simulink model "afe_abc_inv_psm"  (R2025a)
settings: Solver=ode1be  StartTime=0.0  StopTime=simlength  FixedStep=tc  MaxStep=tc
undefined symbols (not defined in the file): Adrso, Amplitude_U, Amplitude_V, Amplitude_W, Aresd, b, Bresd, Cresd, Crso, CTRPIFF_CLIP_RELEASE, dead_time_AFE, dead_time_INV, deepNEGeta, deepNEGxi, deepPOSxi, emf_fb_p, emf_fb_p_ccaller_1, emf_fb_p_ccaller_2, emf_p, emf_p_ccaller_1, emf_p_ccaller_2, end_time_LVRT, fPWM_AFE, fPWM_INV, g0_161Hz, g0_500Hz, g1_161Hz, g1_500Hz, i_grid_neg_eta_lim, i_grid_neg_eta_red_lim, i_grid_neg_xi_lim, i_grid_neg_xi_red_lim, i_grid_pos_eta_lim, i_grid_pos_eta_red_lim, ibez, id_lim, ieta_neg_ref_lim, ieta_pos_ref_lim, Igrid_phase_normalization_factor, iq_lim, ixi_pos_ref_lim, Jm, k_frt_ref, kg, ki_afe, ki_i, ki_rc_neg_grid, ki_rc_pos_grid, ki_vs, ki_w, kp_afe, kp_i, kp_rc_neg_grid, kp_rc_pos_grid, kp_vs, kp_w, kw, l1, l2, Ld_norm ... (+47)
libraries: fl_lib x121, nesl_utility x78, cstblocks x14, simulink x13, single_phase_transformer_lib x3, threephase_inductor_lib x2, flexshaft_lib x1, pmsm_uvw_with_harmonics_lib x1
(part 5 of 10)

== system afe_abc_inv_psm/afe_abc_inv_psm_mod1/afe_control/grid_current_sampling_and_alpha_beta_transformation/sample_hold_normalization ==
  ig_a : Inport
  ig_b : Inport  Port=2
  ig_c : Inport  Port=3
  Gain : Gain  Gain=1/Igrid_phase_normalization_factor
  Gain1 : Gain  Gain=1/Igrid_phase_normalization_factor
  Gain2 : Gain  Gain=1/Igrid_phase_normalization_factor
  Quantizer : Quantizer  QuantizationInterval=adc_quantization
  Quantizer1 : Quantizer  QuantizationInterval=adc_quantization
  Quantizer2 : Quantizer  QuantizationInterval=adc_quantization
  Unit Delay : UnitDelay  SampleTime=ts_afe  HasFrameUpgradeWarning=on
  Unit Delay1 : UnitDelay  SampleTime=ts_afe  HasFrameUpgradeWarning=on
  Unit Delay2 : UnitDelay  SampleTime=ts_afe  HasFrameUpgradeWarning=on
  Zero-Order Hold : ZeroOrderHold  SampleTime=ts_afe
  Zero-Order Hold1 : ZeroOrderHold  SampleTime=ts_afe
  Zero-Order Hold2 : ZeroOrderHold  SampleTime=ts_afe
  ig_a_pu : Outport
  ig_b_pu : Outport  Port=2
  ig_c_pu : Outport  Port=3
  wires:
  ig_a/1 -> Gain/1
  Zero-Order Hold/1 -> Unit Delay/1
  ig_c/1 -> Gain2/1
  ig_b/1 -> Gain1/1
  Unit Delay/1 -> ig_a_pu/1
  Unit Delay1/1 -> ig_b_pu/1
  Unit Delay2/1 -> ig_c_pu/1
  Zero-Order Hold1/1 -> Unit Delay1/1
  Zero-Order Hold2/1 -> Unit Delay2/1
  Quantizer/1 -> Zero-Order Hold/1
  Gain1/1 -> Quantizer1/1
  Gain2/1 -> Quantizer2/1
  Gain/1 -> Quantizer/1
  Quantizer1/1 -> Zero-Order Hold1/1
  Quantizer2/1 -> Zero-Order Hold2/1

== system afe_abc_inv_psm/afe_abc_inv_psm_mod1/afe_control/grid_voltage_phase_lock_loops/DDSRF-PLL ==
  pll_stageA : Subsystem
  pll_stageB : Subsystem
  gamma_grid_ddsrf_pll : Outport
  omega_grid_ddsrf_pll : Outport  Port=2
  wires:
  pll_stageB/1(gamma_grid_ddsrf_pll) -> pll_stageA/1(gamma_grid), gamma_grid_ddsrf_pll/1
  pll_stageA/2(u_grid_pos_eta) -> pll_stageB/2(u_grid_pos_eta)  "u_grid_pos_eta"
  pll_stageA/1(u_grid_pos_xi) -> pll_stageB/1(u_grid_pos_xi)  "u_grid_pos_xi"
  pll_stageB/2(omega_grid_ddsrf_pll) -> omega_grid_ddsrf_pll/1

== system afe_abc_inv_psm/afe_abc_inv_psm_mod1/afe_control/grid_voltage_phase_lock_loops/DQ-PLL ==
  pll_stageA : Subsystem
  pll_stageB : Subsystem
  gamma_grid_dqpll : Outport
  omega_grid_dqpll : Outport  Port=2
  wires:
  pll_stageA/2(u_grid_pos_eta) -> pll_stageB/2(u_grid_pos_eta)  "u_grid_pos_eta"
  pll_stageB/1(gamma_grid_dqpll) -> pll_stageA/1(gamma_grid), gamma_grid_dqpll/1
  pll_stageA/1(u_grid_pos_xi) -> pll_stageB/1(u_grid_pos_xi)  "u_grid_pos_xi"
  pll_stageB/2(omega_grid_dqpll) -> omega_grid_dqpll/1

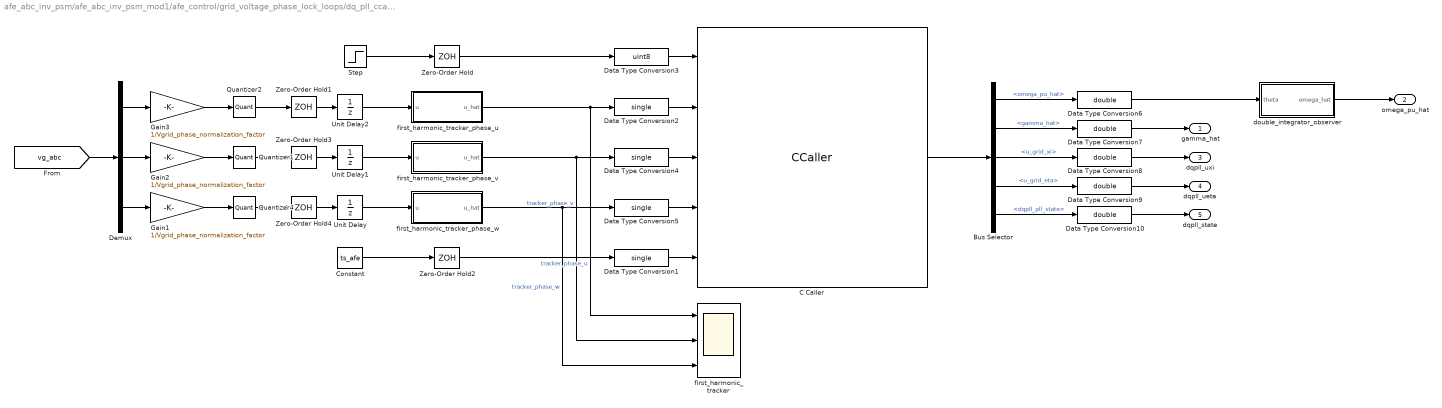
== system afe_abc_inv_psm/afe_abc_inv_psm_mod1/afe_control/grid_voltage_phase_lock_loops/dq_pll_ccaller ==
  Bus Selector : BusSelector  OutputSignals=omega_pu_hat,gamma_hat,u_grid_xi,u_grid_eta,dqpll_pll_state
  C Caller : CCaller  FunctionName=dqpll_grid_process_simulink  PortSpecificationStruct="%)30     .    N H   8    (     @         %    \"     8    !     0         %  0 \"0    $    _    07)G3F%M90  4&]R=$YA;64 4V-O<&4     26YD97@     5'EP90      4VEZ90      27-';&]B86P   X    P    !@    @    $          4    (     0    ,    !         !   P!O=70 #@   #     &    \"     0         !0    @    !     P    $         $  # &]U=  .    .     8    (    !          %    \"     $    &     0         0   ...(+3319 chars)"  SampleTime=ts_afe
  Constant : Constant  Value=ts_afe
  Data Type Conversion{1..2,4..5} (4 alike) : DataTypeConversion  OutDataTypeStr=single  SaturateOnIntegerOverflow=off  RndMeth=Floor
  Data Type Conversion{6..10} (5 alike) : DataTypeConversion  OutDataTypeStr=double  SaturateOnIntegerOverflow=off  RndMeth=Floor
  Data Type Conversion3 : DataTypeConversion  OutDataTypeStr=uint8  SaturateOnIntegerOverflow=off  RndMeth=Floor
  Demux : Demux  Outputs=3
  Gain1 : Gain  Gain=1/Vgrid_phase_normalization_factor
  Gain2 : Gain  Gain=1/Vgrid_phase_normalization_factor
  Gain3 : Gain  Gain=1/Vgrid_phase_normalization_factor
  Quantizer1 : Quantizer  QuantizationInterval=adc_quantization
  Quantizer2 : Quantizer  QuantizationInterval=adc_quantization
  Quantizer4 : Quantizer  QuantizationInterval=adc_quantization
  Step : Step  Time=0.01  Before=1  After=0  SampleTime=0
  Unit Delay : UnitDelay  SampleTime=ts_afe  HasFrameUpgradeWarning=on
  Unit Delay1 : UnitDelay  SampleTime=ts_afe  HasFrameUpgradeWarning=on
  Unit Delay2 : UnitDelay  SampleTime=ts_afe  HasFrameUpgradeWarning=on
  Zero-Order Hold : ZeroOrderHold  SampleTime=ts_afe
  Zero-Order Hold1 : ZeroOrderHold  SampleTime=-1
  Zero-Order Hold2 : ZeroOrderHold  SampleTime=ts_afe
  Zero-Order Hold3 : ZeroOrderHold  SampleTime=-1
  Zero-Order Hold4 : ZeroOrderHold  SampleTime=-1
  double_integrator_observer : Subsystem
  first_harmonic_tracker : Scope  NumInputPorts=3
      settings: SampleTime=ts_afe  ActiveDisplayYMinimum=-1.8038768619298935  ActiveDisplayYMaximum=1.5708545297384262
  first_harmonic_tracker_phase_u : Subsystem
  first_harmonic_tracker_phase_v : Subsystem
  first_harmonic_tracker_phase_w : Subsystem
  gamma_hat : Outport  VectorParamsAs1DForOutWhenUnconnected=off
  omega_pu_hat : Outport  Port=2  VectorParamsAs1DForOutWhenUnconnected=off
  dqpll_uxi : Outport  Port=3  VectorParamsAs1DForOutWhenUnconnected=off
  dqpll_ueta : Outport  Port=4  VectorParamsAs1DForOutWhenUnconnected=off
  dqpll_state : Outport  Port=5  VectorParamsAs1DForOutWhenUnconnected=off
  wires:
  Zero-Order Hold/1 -> Data Type Conversion3/1
  Step/1 -> Zero-Order Hold/1
  Zero-Order Hold2/1 -> Data Type Conversion1/1
  Constant/1 -> Zero-Order Hold2/1
  Data Type Conversion3/1 -> C Caller/1
  Data Type Conversion2/1 -> C Caller/2
  Data Type Conversion4/1 -> C Caller/3
  Data Type Conversion5/1 -> C Caller/4
  Data Type Conversion1/1 -> C Caller/5
  C Caller/1 -> Bus Selector/1
  Bus Selector/1 -> Data Type Conversion6/1  "<omega_pu_hat>"
  Bus Selector/2 -> Data Type Conversion7/1  "<gamma_hat>"
  Bus Selector/3 -> Data Type Conversion8/1  "<u_grid_xi>"
  Bus Selector/4 -> Data Type Conversion9/1  "<u_grid_eta>"
  Bus Selector/5 -> Data Type Conversion10/1  "<dqpll_pll_state>"
  Data Type Conversion6/1 -> double_integrator_observer/1(theta)
  Data Type Conversion7/1 -> gamma_hat/1
  Data Type Conversion10/1 -> dqpll_state/1
  Data Type Conversion8/1 -> dqpll_uxi/1
  Data Type Conversion9/1 -> dqpll_ueta/1
  [vg_abc] -> Demux/1
  Quantizer4/1 -> Zero-Order Hold4/1
  Quantizer2/1 -> Zero-Order Hold1/1
  Gain2/1 -> Quantizer1/1
  Gain3/1 -> Quantizer2/1
  Gain1/1 -> Quantizer4/1
  Zero-Order Hold1/1 -> Unit Delay2/1
  Unit Delay2/1 -> first_harmonic_tracker_phase_u/1(u)
  Demux/1 -> Gain3/1
  Unit Delay1/1 -> first_harmonic_tracker_phase_v/1(u)
  Demux/2 -> Gain2/1
  Demux/3 -> Gain1/1
  Unit Delay/1 -> first_harmonic_tracker_phase_w/1(u)
  Quantizer1/1 -> Zero-Order Hold3/1
  Zero-Order Hold3/1 -> Unit Delay1/1
  Zero-Order Hold4/1 -> Unit Delay/1
  double_integrator_observer/1(omega_hat) -> omega_pu_hat/1
  first_harmonic_tracker_phase_u/1(u_hat) -> first_harmonic_tracker/1, Data Type Conversion2/1  "tracker_phase_u"
  first_harmonic_tracker_phase_v/1(u_hat) -> first_harmonic_tracker/2, Data Type Conversion4/1  "tracker_phase_v"
  first_harmonic_tracker_phase_w/1(u_hat) -> first_harmonic_tracker/3, Data Type Conversion5/1  "tracker_phase_w"

== system afe_abc_inv_psm/afe_abc_inv_psm_mod1/afe_control/grid_voltage_sampling_and_alpha_beta_transformation/sample_hold_normalization ==
  vg_a : Inport
  vg_b : Inport  Port=2
  vg_c : Inport  Port=3
  Gain : Gain  Gain=1/Vgrid_phase_normalization_factor
  Gain1 : Gain  Gain=1/Vgrid_phase_normalization_factor
  Gain2 : Gain  Gain=1/Vgrid_phase_normalization_factor
  Quantizer1 : Quantizer  QuantizationInterval=adc_quantization
  Quantizer2 : Quantizer  QuantizationInterval=adc_quantization
  Quantizer3 : Quantizer  QuantizationInterval=adc_quantization
  Unit Delay : UnitDelay  SampleTime=ts_afe  HasFrameUpgradeWarning=on
  Unit Delay1 : UnitDelay  SampleTime=ts_afe  HasFrameUpgradeWarning=on
  Unit Delay2 : UnitDelay  SampleTime=ts_afe  HasFrameUpgradeWarning=on
  Zero-Order Hold : ZeroOrderHold  SampleTime=ts_afe
  Zero-Order Hold1 : ZeroOrderHold  SampleTime=ts_afe
  Zero-Order Hold2 : ZeroOrderHold  SampleTime=ts_afe
  vg_a_pu : Outport
  vg_b_pu : Outport  Port=2
  vg_c_pu : Outport  Port=3
  wires:
  vg_a/1 -> Gain/1
  Zero-Order Hold/1 -> Unit Delay/1
  vg_c/1 -> Gain2/1
  vg_b/1 -> Gain1/1
  Unit Delay/1 -> vg_a_pu/1
  Unit Delay1/1 -> vg_b_pu/1
  Unit Delay2/1 -> vg_c_pu/1
  Zero-Order Hold1/1 -> Unit Delay1/1
  Zero-Order Hold2/1 -> Unit Delay2/1
  Quantizer1/1 -> Zero-Order Hold/1
  Gain1/1 -> Quantizer2/1
  Gain2/1 -> Quantizer3/1
  Gain/1 -> Quantizer1/1
  Quantizer2/1 -> Zero-Order Hold1/1
  Quantizer3/1 -> Zero-Order Hold2/1

== system afe_abc_inv_psm/afe_abc_inv_psm_mod1/afe_control/islanding_mode_detector/Moving Average Filter ==
  u_7th : Inport
  In3 : Inport  Port=2
  Bus Selector : BusSelector  OutputSignals=ts,sshort,slong,pinput,cbpointer,cbsample,mavg_output
  C Caller : CCaller  FunctionName=mavgflt_process_simulink  PortSpecificationStruct="%)30     .    B H   8    (     @         %    \"     8    !     0         %  0 \"0    $    _    07)G3F%M90  4&]R=$YA;64 4V-O<&4     26YD97@     5'EP90      4VEZ90      27-';&]B86P   X    P    !@    @    $          4    (     0    ,    !         !   P!O=70 #@   #     &    \"     0         !0    @    !     P    $         $  # &]U=  .    .     8    (    !          %    \"     $    &     0         0   ...(+3251 chars)"  SampleTime=ts_afe
  Compare To Zero : simulink/Logic and Bit Operations/Compare To Zero  relop=>  OutDataTypeStr=boolean
  Constant : Constant  Value=9
  Constant5 : Constant  Value=ts_afe
  Data Type Conversion : DataTypeConversion  OutDataTypeStr=single  SaturateOnIntegerOverflow=off  RndMeth=Floor
  Data Type Conversion1 : DataTypeConversion  OutDataTypeStr=single  SaturateOnIntegerOverflow=off  RndMeth=Floor
  Data Type Conversion2 : DataTypeConversion  OutDataTypeStr=single  SaturateOnIntegerOverflow=off  RndMeth=Floor
  Data Type Conversion3 : DataTypeConversion  OutDataTypeStr=double  SaturateOnIntegerOverflow=off  RndMeth=Floor
  Data Type Conversion4 : DataTypeConversion  OutDataTypeStr=uint8  SaturateOnIntegerOverflow=off  RndMeth=Floor
  Data Type Conversion5 : DataTypeConversion  OutDataTypeStr=uint8  SaturateOnIntegerOverflow=off  RndMeth=Floor
  Enabled Subsystem : Subsystem  TreatAsAtomicUnit=on
  Reset Trigger : Subsystem
  Terminator{,1..5} (6 alike) : Terminator
  Zero-Order Hold1 : ZeroOrderHold  SampleTime=ts_afe
  Zero-Order Hold2 : ZeroOrderHold  SampleTime=ts_afe
  xi : Outport
  wires:
  Bus Selector/5 -> Terminator2/1  "<cbpointer>"
  Bus Selector/4 -> Terminator1/1  "<pinput>"
  Data Type Conversion3/1 -> xi/1  "output"
  Zero-Order Hold2/1 -> Data Type Conversion/1  "d1"
  Enabled Subsystem/1(Out1) -> Data Type Conversion1/1
  Compare To Zero/1 -> Enabled Subsystem/Enable
  In3/1 -> Enabled Subsystem/1(In1), Compare To Zero/1  "omega_grid"
  Constant5/1 -> Zero-Order Hold1/1
  Zero-Order Hold1/1 -> Data Type Conversion2/1  "d1"
  Bus Selector/3 -> Terminator4/1  "<slong>"
  Bus Selector/2 -> Terminator3/1  "<sshort>"
  Bus Selector/1 -> Terminator/1  "<ts>"
  C Caller/1 -> Bus Selector/1  "out"
  u_7th/1 -> Zero-Order Hold2/1  "input"
  Data Type Conversion4/1 -> C Caller/5
  Data Type Conversion/1 -> C Caller/1  "input"
  Data Type Conversion5/1 -> C Caller/4
  Data Type Conversion2/1 -> C Caller/3
  Data Type Conversion1/1 -> C Caller/2
  Reset Trigger/1(Out1) -> Data Type Conversion5/1
  Constant/1 -> Data Type Conversion4/1
  Bus Selector/6 -> Terminator5/1  "<cbsample>"
  Bus Selector/7 -> Data Type Conversion3/1  "<mavg_output>"

== system afe_abc_inv_psm/afe_abc_inv_psm_mod1/afe_control/islanding_mode_detector/Moving Average Filter1 ==
  u_7th : Inport
  In3 : Inport  Port=2
  Bus Selector : BusSelector  OutputSignals=ts,sshort,slong,pinput,cbpointer,cbsample,mavg_output
  C Caller : CCaller  FunctionName=mavgflt_process_simulink  PortSpecificationStruct="%)30     .    B H   8    (     @         %    \"     8    !     0         %  0 \"0    $    _    07)G3F%M90  4&]R=$YA;64 4V-O<&4     26YD97@     5'EP90      4VEZ90      27-';&]B86P   X    P    !@    @    $          4    (     0    ,    !         !   P!O=70 #@   #     &    \"     0         !0    @    !     P    $         $  # &]U=  .    .     8    (    !          %    \"     $    &     0         0   ...(+3251 chars)"  SampleTime=ts_afe
  Compare To Zero : simulink/Logic and Bit Operations/Compare To Zero  relop=>  OutDataTypeStr=boolean
  Constant : Constant  Value=10
  Constant5 : Constant  Value=ts_afe
  Data Type Conversion : DataTypeConversion  OutDataTypeStr=single  SaturateOnIntegerOverflow=off  RndMeth=Floor
  Data Type Conversion1 : DataTypeConversion  OutDataTypeStr=single  SaturateOnIntegerOverflow=off  RndMeth=Floor
  Data Type Conversion2 : DataTypeConversion  OutDataTypeStr=single  SaturateOnIntegerOverflow=off  RndMeth=Floor
  Data Type Conversion3 : DataTypeConversion  OutDataTypeStr=double  SaturateOnIntegerOverflow=off  RndMeth=Floor
  Data Type Conversion4 : DataTypeConversion  OutDataTypeStr=uint8  SaturateOnIntegerOverflow=off  RndMeth=Floor
  Data Type Conversion5 : DataTypeConversion  OutDataTypeStr=uint8  SaturateOnIntegerOverflow=off  RndMeth=Floor
  Enabled Subsystem : Subsystem  TreatAsAtomicUnit=on
  Reset Trigger : Subsystem
  Terminator{,1..5} (6 alike) : Terminator
  Zero-Order Hold1 : ZeroOrderHold  SampleTime=ts_afe
  Zero-Order Hold2 : ZeroOrderHold  SampleTime=ts_afe
  xi : Outport
  wires:
  Bus Selector/7 -> Data Type Conversion3/1  "<mavg_output>"
  Bus Selector/6 -> Terminator5/1  "<cbsample>"
  Constant/1 -> Data Type Conversion4/1
  Reset Trigger/1(Out1) -> Data Type Conversion5/1
  Data Type Conversion1/1 -> C Caller/2
  Data Type Conversion2/1 -> C Caller/3
  Data Type Conversion5/1 -> C Caller/4
  Data Type Conversion/1 -> C Caller/1  "input"
  Data Type Conversion4/1 -> C Caller/5
  u_7th/1 -> Zero-Order Hold2/1  "input"
  C Caller/1 -> Bus Selector/1  "out"
  Bus Selector/1 -> Terminator/1  "<ts>"
  Bus Selector/2 -> Terminator3/1  "<sshort>"
  Bus Selector/3 -> Terminator4/1  "<slong>"
  Zero-Order Hold1/1 -> Data Type Conversion2/1  "d1"
  Constant5/1 -> Zero-Order Hold1/1
  In3/1 -> Compare To Zero/1, Enabled Subsystem/1(In1)  "omega_grid"
  Compare To Zero/1 -> Enabled Subsystem/Enable
  Enabled Subsystem/1(Out1) -> Data Type Conversion1/1
  Zero-Order Hold2/1 -> Data Type Conversion/1  "d1"
  Data Type Conversion3/1 -> xi/1  "output"
  Bus Selector/4 -> Terminator1/1  "<pinput>"
  Bus Selector/5 -> Terminator2/1  "<cbpointer>"

== system afe_abc_inv_psm/afe_abc_inv_psm_mod1/afe_control/sequences_current_control/Negative-Seq. eta-Control ==
  ff : Inport
  e : Inport  Port=2
  1/Ti : Gain  Gain=kp_rc_neg_grid  SaturateOnIntegerOverflow=on  OutDataTypeStr=Inherit: Same as input  ParamDataTypeStr=Inherit: Same as input
  1/Ti1 : Gain  SaturateOnIntegerOverflow=on  OutDataTypeStr=Inherit: Same as input  ParamDataTypeStr=Inherit: Same as input
  Saturation : Saturate  UpperLimit=ieta_neg_ref_lim  LowerLimit=-ieta_neg_ref_lim
  Sum : Sum  Inputs=|++
  Sum2 : Sum  Inputs=+++  SaturateOnIntegerOverflow=on
  Sum3 : Sum  Inputs=-+  SaturateOnIntegerOverflow=on
  Unit Delay4 : UnitDelay  SampleTime=ts_afe  HasFrameUpgradeWarning=on
  kp : Gain  Gain=ki_rc_neg_grid*ts_afe  SaturateOnIntegerOverflow=on  OutDataTypeStr=Inherit: Same as input  ParamDataTypeStr=Inherit: Same as input
  u : Outport  VectorParamsAs1DForOutWhenUnconnected=off
  wires:
  Unit Delay4/1 -> Sum2/3
  Sum3/1 -> Unit Delay4/1
  kp/1 -> Sum2/2
  Sum2/1 -> Saturation/1
  1/Ti/1 -> Sum2/1, Sum3/1
  Saturation/1 -> Sum/1, Sum3/2
  Sum/1 -> u/1
  ff/1 -> 1/Ti1/1
  1/Ti1/1 -> Sum/2
  e/1 -> 1/Ti/1, kp/1  "e"

== system afe_abc_inv_psm/afe_abc_inv_psm_mod1/afe_control/sequences_current_control/Negative-Seq. xi-Control ==
  ff : Inport
  e : Inport  Port=2
  1/Ti : Gain  Gain=kp_rc_neg_grid  SaturateOnIntegerOverflow=on  OutDataTypeStr=Inherit: Same as input  ParamDataTypeStr=Inherit: Same as input
  1/Ti1 : Gain  SaturateOnIntegerOverflow=on  OutDataTypeStr=Inherit: Same as input  ParamDataTypeStr=Inherit: Same as input
  Saturation : Saturate  UpperLimit=ieta_pos_ref_lim  LowerLimit=-ieta_pos_ref_lim
  Sum : Sum  Inputs=|++
  Sum2 : Sum  Inputs=+++  SaturateOnIntegerOverflow=on
  Sum3 : Sum  Inputs=-+  SaturateOnIntegerOverflow=on
  Unit Delay4 : UnitDelay  SampleTime=ts_afe  HasFrameUpgradeWarning=on
  kp : Gain  Gain=ki_rc_neg_grid*ts_afe  SaturateOnIntegerOverflow=on  OutDataTypeStr=Inherit: Same as input  ParamDataTypeStr=Inherit: Same as input
  u : Outport  VectorParamsAs1DForOutWhenUnconnected=off
  wires:
  Unit Delay4/1 -> Sum2/3
  Sum3/1 -> Unit Delay4/1
  kp/1 -> Sum2/2
  Sum2/1 -> Saturation/1
  1/Ti/1 -> Sum2/1, Sum3/1
  Saturation/1 -> Sum/1, Sum3/2
  Sum/1 -> u/1
  ff/1 -> 1/Ti1/1
  1/Ti1/1 -> Sum/2
  e/1 -> 1/Ti/1, kp/1  "e"

== system afe_abc_inv_psm/afe_abc_inv_psm_mod1/afe_control/sequences_current_control/Positive-Seq. eta-Control ==
  ff : Inport
  e : Inport  Port=2
  1/Ti : Gain  Gain=kp_rc_pos_grid  SaturateOnIntegerOverflow=on  OutDataTypeStr=Inherit: Same as input  ParamDataTypeStr=Inherit: Same as input
  1/Ti1 : Gain  SaturateOnIntegerOverflow=on  OutDataTypeStr=Inherit: Same as input  ParamDataTypeStr=Inherit: Same as input
  Saturation : Saturate  UpperLimit=ieta_pos_ref_lim  LowerLimit=-ieta_pos_ref_lim
  Sum : Sum  Inputs=|++
  Sum2 : Sum  Inputs=+++  SaturateOnIntegerOverflow=on
  Sum3 : Sum  Inputs=-+  SaturateOnIntegerOverflow=on
  Unit Delay4 : UnitDelay  SampleTime=ts_afe  HasFrameUpgradeWarning=on
  kp : Gain  Gain=ki_rc_pos_grid*ts_afe  SaturateOnIntegerOverflow=on  OutDataTypeStr=Inherit: Same as input  ParamDataTypeStr=Inherit: Same as input
  u : Outport  VectorParamsAs1DForOutWhenUnconnected=off
  wires:
  Unit Delay4/1 -> Sum2/3
  Sum3/1 -> Unit Delay4/1
  kp/1 -> Sum2/2
  Sum2/1 -> Saturation/1
  1/Ti/1 -> Sum2/1, Sum3/1
  Saturation/1 -> Sum/1, Sum3/2
  Sum/1 -> u/1
  ff/1 -> 1/Ti1/1
  1/Ti1/1 -> Sum/2
  e/1 -> 1/Ti/1, kp/1  "e"

== system afe_abc_inv_psm/afe_abc_inv_psm_mod1/afe_control/voltage_sequence_avg/average_filter_ccaller ==
  v_grid_pos_xi : Inport
  v_grid_pos_eta : Inport  Port=2
  v_grid_neg_xi : Inport  Port=3
  v_grid_neg_eta : Inport  Port=4
  Moving Average Filter1 : Subsystem
  Moving Average Filter2 : Subsystem
  Moving Average Filter3 : Subsystem
  Moving Average Filter4 : Subsystem
  v_grid_pos_xi_avg : Outport
  v_grid_pos_eta_avg : Outport  Port=2
  v_grid_neg_xi_avg : Outport  Port=3
  v_grid_neg_eta_avg : Outport  Port=4
  wires:
  Moving Average Filter2/1(xi) -> v_grid_pos_eta_avg/1
  [omega_grid_pll] -> Moving Average Filter1/2(In3), Moving Average Filter2/2(In3), Moving Average Filter4/2(In3), Moving Average Filter3/2(In3)
  v_grid_pos_xi/1 -> Moving Average Filter1/1(In2)
  v_grid_neg_xi/1 -> Moving Average Filter3/1(In2)
  v_grid_neg_eta/1 -> Moving Average Filter4/1(In2)
  Moving Average Filter3/1(xi) -> v_grid_neg_xi_avg/1
  Moving Average Filter4/1(xi) -> v_grid_neg_eta_avg/1
  Moving Average Filter1/1(xi) -> v_grid_pos_xi_avg/1
  v_grid_pos_eta/1 -> Moving Average Filter2/1(In2)

== system afe_abc_inv_psm/afe_abc_inv_psm_mod1/afe_control/voltage_sequence_avg/average_filter_simulink ==
  v_grid_pos_xi : Inport
  v_grid_pos_eta : Inport  Port=2
  v_grid_neg_xi : Inport  Port=3
  v_grid_neg_eta : Inport  Port=4
  mavg_1 : Subsystem
  mavg_2 : Subsystem
  mavg_3 : Subsystem
  mavg_4 : Subsystem
  v_grid_pos_xi_avg : Outport
  v_grid_pos_eta_avg : Outport  Port=2
  v_grid_neg_xi_avg : Outport  Port=3
  v_grid_neg_eta_avg : Outport  Port=4
  wires:
  mavg_3/1(out) -> v_grid_neg_xi_avg/1
  mavg_1/1(out) -> v_grid_pos_xi_avg/1
  v_grid_pos_eta/1 -> mavg_2/1(in)
  v_grid_neg_eta/1 -> mavg_4/1(in)
  v_grid_pos_xi/1 -> mavg_1/1(in)
  mavg_4/1(out) -> v_grid_neg_eta_avg/1
  v_grid_neg_xi/1 -> mavg_3/1(in)
  mavg_2/1(out) -> v_grid_pos_eta_avg/1

== system afe_abc_inv_psm/afe_abc_inv_psm_mod1/inverter/inverter/sv_pwm ==
  ab : Inport
  enable : Inport  Port=2
  Bus Selector : BusSelector  OutputSignals=da,db,dc
  Bus Selector1 : BusSelector  OutputSignals=ua,ub
  C Caller : CCaller  FunctionName=sv_pwm_process_simulink  PortSpecificationStruct="%)30     .    V @   8    (     @         %    \"     4    !     0         %  0 \"0    $    _    07)G3F%M90  4&]R=$YA;64 4V-O<&4     26YD97@     5'EP90      4VEZ90      27-';&]B86P   X    P    !@    @    $          4    (     0    ,    !         !   P!O=70 #@   #     &    \"     0         !0    @    !     P    $         $  # &]U=  .    .     8    (    !          %    \"     $    &     0         0   ...(+2669 chars)"  SampleTime=ts_inv
  Constant : Constant  Value=ts_inv
  Data Type Conversion1 : DataTypeConversion  OutDataTypeStr=double  SaturateOnIntegerOverflow=off  RndMeth=Floor
  Data Type Conversion15 : DataTypeConversion  OutDataTypeStr=single  SaturateOnIntegerOverflow=off  RndMeth=Floor
  Data Type Conversion16 : DataTypeConversion  OutDataTypeStr=single  SaturateOnIntegerOverflow=off  RndMeth=Floor
  Data Type Conversion17 : DataTypeConversion  OutDataTypeStr=uint32  SaturateOnIntegerOverflow=off  RndMeth=Floor
  Data Type Conversion18 : DataTypeConversion  OutDataTypeStr=single  SaturateOnIntegerOverflow=off  RndMeth=Floor
  Data Type Conversion2 : DataTypeConversion  OutDataTypeStr=double  SaturateOnIntegerOverflow=off  RndMeth=Floor
  Data Type Conversion3 : DataTypeConversion  OutDataTypeStr=double  SaturateOnIntegerOverflow=off  RndMeth=Floor
  Zero-Order Hold{,1..3} (4 alike) : ZeroOrderHold  SampleTime=ts_afe
  modulator1 : Subsystem
  firing_gates : Outport
  wires:
  Data Type Conversion1/1 -> modulator1/1(u)  "du"
  Zero-Order Hold/1 -> C Caller/1
  Zero-Order Hold2/1 -> C Caller/3
  Constant/1 -> Data Type Conversion16/1
  Data Type Conversion18/1 -> Zero-Order Hold/1
  enable/1 -> Data Type Conversion17/1
  Data Type Conversion2/1 -> modulator1/2(v)  "dv"
  Data Type Conversion16/1 -> Zero-Order Hold2/1
  Zero-Order Hold1/1 -> C Caller/2
  Data Type Conversion17/1 -> Zero-Order Hold3/1
  Zero-Order Hold3/1 -> C Caller/4
  Data Type Conversion15/1 -> Zero-Order Hold1/1
  C Caller/1 -> Bus Selector/1  "out"
  Data Type Conversion3/1 -> modulator1/3(w)  "dw"
  modulator1/1(cmd_gates) -> firing_gates/1
  ab/1 -> Bus Selector1/1
  Bus Selector1/1 -> Data Type Conversion18/1  "<ua>"
  Bus Selector1/2 -> Data Type Conversion15/1  "<ub>"
  Bus Selector/1 -> Data Type Conversion1/1  "<da>"
  Bus Selector/3 -> Data Type Conversion3/1  "<dc>"
  Bus Selector/2 -> Data Type Conversion2/1  "<db>"

== system afe_abc_inv_psm/afe_abc_inv_psm_mod1/inverter/inverter/switch_1 ==
  Diode : fl_lib/Electrical/Electrical Elements/Diode  Vf=Vgamma V  Ron=Ron Ohm  Goff=1e-8 1/Ohm  i_specify=off  i_priority=None  i=0 A  i_nominal_specify=off  i_nominal_value=1  i_nominal_unit=A  v_specify=off  v_priority=None  v=0 V  v_nominal_specify=off  v_nominal_value=1  v_nominal_unit=V
  Switch : fl_lib/Electrical/Electrical Elements/Switch  R_closed=Ron Ohm  G_open=1e-8 1/Ohm  Threshold=7.5  i_specify=off  i_priority=None  i=0 A  i_nominal_specify=off  i_nominal_value=1  i_nominal_unit=A  v_specify=off  v_priority=None  v=0 V  v_nominal_specify=off  v_nominal_value=1  v_nominal_unit=V
  G : PMIOPort  Side=Left
  C : PMIOPort  Port=2  Side=Left
  E : PMIOPort  Port=3  Side=Right
  connections:
  Switch/RConn2 -- C/RConn1 -- Diode/RConn1
  Switch/RConn1 -- G/RConn1
  Switch/LConn1 -- E/RConn1 -- Diode/LConn1

== system afe_abc_inv_psm/afe_abc_inv_psm_mod1/inverter/inverter/switch_2 ==
  Diode : fl_lib/Electrical/Electrical Elements/Diode  Vf=Vgamma V  Ron=Ron Ohm  Goff=1e-8 1/Ohm  i_specify=off  i_priority=None  i=0 A  i_nominal_specify=off  i_nominal_value=1  i_nominal_unit=A  v_specify=off  v_priority=None  v=0 V  v_nominal_specify=off  v_nominal_value=1  v_nominal_unit=V
  Switch : fl_lib/Electrical/Electrical Elements/Switch  R_closed=Ron Ohm  G_open=1e-8 1/Ohm  Threshold=7.5  i_specify=off  i_priority=None  i=0 A  i_nominal_specify=off  i_nominal_value=1  i_nominal_unit=A  v_specify=off  v_priority=None  v=0 V  v_nominal_specify=off  v_nominal_value=1  v_nominal_unit=V
  G : PMIOPort  Side=Left
  C : PMIOPort  Port=2  Side=Left
  E : PMIOPort  Port=3  Side=Right
  connections:
  Diode/LConn1 -- E/RConn1 -- Switch/LConn1
  Switch/RConn1 -- G/RConn1
  Diode/RConn1 -- C/RConn1 -- Switch/RConn2

== system afe_abc_inv_psm/afe_abc_inv_psm_mod1/inverter/inverter/switch_3 ==
  Diode : fl_lib/Electrical/Electrical Elements/Diode  Vf=Vgamma V  Ron=Ron Ohm  Goff=1e-8 1/Ohm  i_specify=off  i_priority=None  i=0 A  i_nominal_specify=off  i_nominal_value=1  i_nominal_unit=A  v_specify=off  v_priority=None  v=0 V  v_nominal_specify=off  v_nominal_value=1  v_nominal_unit=V
  Switch : fl_lib/Electrical/Electrical Elements/Switch  R_closed=Ron Ohm  G_open=1e-8 1/Ohm  Threshold=7.5  i_specify=off  i_priority=None  i=0 A  i_nominal_specify=off  i_nominal_value=1  i_nominal_unit=A  v_specify=off  v_priority=None  v=0 V  v_nominal_specify=off  v_nominal_value=1  v_nominal_unit=V
  G : PMIOPort  Side=Left
  C : PMIOPort  Port=2  Side=Left
  E : PMIOPort  Port=3  Side=Right
  connections:
  Diode/LConn1 -- E/RConn1 -- Switch/LConn1
  Switch/RConn1 -- G/RConn1
  Diode/RConn1 -- C/RConn1 -- Switch/RConn2

== system afe_abc_inv_psm/afe_abc_inv_psm_mod1/inverter/inverter/switch_4 ==
  Diode : fl_lib/Electrical/Electrical Elements/Diode  Vf=Vgamma V  Ron=Ron Ohm  Goff=1e-8 1/Ohm  i_specify=off  i_priority=None  i=0 A  i_nominal_specify=off  i_nominal_value=1  i_nominal_unit=A  v_specify=off  v_priority=None  v=0 V  v_nominal_specify=off  v_nominal_value=1  v_nominal_unit=V
  Switch : fl_lib/Electrical/Electrical Elements/Switch  R_closed=Ron Ohm  G_open=1e-8 1/Ohm  Threshold=7.5  i_specify=off  i_priority=None  i=0 A  i_nominal_specify=off  i_nominal_value=1  i_nominal_unit=A  v_specify=off  v_priority=None  v=0 V  v_nominal_specify=off  v_nominal_value=1  v_nominal_unit=V
  G : PMIOPort  Side=Left
  C : PMIOPort  Port=2  Side=Left
  E : PMIOPort  Port=3  Side=Right
  connections:
  Switch/RConn2 -- C/RConn1 -- Diode/RConn1
  Switch/RConn1 -- G/RConn1
  Switch/LConn1 -- E/RConn1 -- Diode/LConn1

== system afe_abc_inv_psm/afe_abc_inv_psm_mod1/inverter/inverter/switch_5 ==
  Diode : fl_lib/Electrical/Electrical Elements/Diode  Vf=Vgamma V  Ron=Ron Ohm  Goff=1e-8 1/Ohm  i_specify=off  i_priority=None  i=0 A  i_nominal_specify=off  i_nominal_value=1  i_nominal_unit=A  v_specify=off  v_priority=None  v=0 V  v_nominal_specify=off  v_nominal_value=1  v_nominal_unit=V
  Switch : fl_lib/Electrical/Electrical Elements/Switch  R_closed=Ron Ohm  G_open=1e-8 1/Ohm  Threshold=7.5  i_specify=off  i_priority=None  i=0 A  i_nominal_specify=off  i_nominal_value=1  i_nominal_unit=A  v_specify=off  v_priority=None  v=0 V  v_nominal_specify=off  v_nominal_value=1  v_nominal_unit=V
  G : PMIOPort  Side=Left
  C : PMIOPort  Port=2  Side=Left
  E : PMIOPort  Port=3  Side=Right
  connections:
  Diode/LConn1 -- E/RConn1 -- Switch/LConn1
  Switch/RConn1 -- G/RConn1
  Diode/RConn1 -- C/RConn1 -- Switch/RConn2

== system afe_abc_inv_psm/afe_abc_inv_psm_mod1/inverter/inverter/switch_6 ==
  Diode : fl_lib/Electrical/Electrical Elements/Diode  Vf=Vgamma V  Ron=Ron Ohm  Goff=1e-8 1/Ohm  i_specify=off  i_priority=None  i=0 A  i_nominal_specify=off  i_nominal_value=1  i_nominal_unit=A  v_specify=off  v_priority=None  v=0 V  v_nominal_specify=off  v_nominal_value=1  v_nominal_unit=V
  Switch : fl_lib/Electrical/Electrical Elements/Switch  R_closed=Ron Ohm  G_open=1e-8 1/Ohm  Threshold=7.5  i_specify=off  i_priority=None  i=0 A  i_nominal_specify=off  i_nominal_value=1  i_nominal_unit=A  v_specify=off  v_priority=None  v=0 V  v_nominal_specify=off  v_nominal_value=1  v_nominal_unit=V
  G : PMIOPort  Side=Left
  C : PMIOPort  Port=2  Side=Left
  E : PMIOPort  Port=3  Side=Right
  connections:
  Switch/RConn2 -- C/RConn1 -- Diode/RConn1
  Switch/RConn1 -- G/RConn1
  Switch/LConn1 -- E/RConn1 -- Diode/LConn1

== system afe_abc_inv_psm/afe_abc_inv_psm_mod1/inverter_control/current_ctrl/bemf_observer ==
  ialpha_pu : Inport
  ibeta_pu : Inport  Port=2
  ualpha_pu : Inport  Port=3
  ubeta_pu : Inport  Port=4
  BEMF Observer simulink/Ccaller : Scope  NumInputPorts=2
      settings: SampleTime=tc  ActiveDisplayYMinimum=-1.1712299957043022  ActiveDisplayYMaximum=1.2529884353188021
  Mux : Mux  Inputs=3
  Mux1 : Mux  Inputs=3
  Variant Source : VariantSource  VariantControls={use_observer_from_simulink_module_1 == 1, use_observer_from_ccaller_module_1 == 1}
  Variant Source1 : VariantSource  VariantControls={use_observer_from_simulink_module_1 == 1, use_observer_from_ccaller_module_1 == 1}
  bemf_observer : Subsystem
  bemf_observer_ccaller : Subsystem
  double_integrator_observer : Subsystem
  phase_fault : Subsystem
  tag scope: omega_hat_pu=global, theta_hat=global
  wires:
  ialpha_pu/1 -> bemf_observer/1(ialpha_pu), bemf_observer_ccaller/1(ialpha_pu)
  ibeta_pu/1 -> bemf_observer/2(ibeta_pu), bemf_observer_ccaller/2(ibeta_pu)
  Mux/1 -> BEMF Observer simulink/Ccaller/1
  Mux1/1 -> BEMF Observer simulink/Ccaller/2
  double_integrator_observer/1(omega_pu_hat) -> Mux/3  "omega_pu_encoder"
  ualpha_pu/1 -> bemf_observer/3(ualpha_pu), bemf_observer_ccaller/3(ualpha_pu)
  ubeta_pu/1 -> bemf_observer/4(ubeta_pu), bemf_observer_ccaller/4(ubeta_pu)
  double_integrator_observer/2(theta_hat) -> Mux1/3  "theta_hat_encoder"
  [theta_elec_pmsm] -> phase_fault/1(theta_pmsm)  "theta_pmsm"
  phase_fault/1(theta) -> double_integrator_observer/1(theta)
  bemf_observer/1(omega_pu) -> Mux/1, Variant Source/1  "omega_pu"
  bemf_observer_ccaller/2(theta_hat) -> Mux1/2, Variant Source1/2  "theta_hat_code"
  bemf_observer_ccaller/1(omega_pu) -> Mux/2, Variant Source/2  "omega_pu_code"
  bemf_observer/2(theta_hat) -> Variant Source1/1, Mux1/1  "theta_hat"
  Variant Source1/1 -> [theta_hat]
  Variant Source/1 -> [omega_hat_pu]

== system afe_abc_inv_psm/afe_abc_inv_psm_mod1/inverter_control/current_ctrl/current_ctrl ==
  iq_ref : Inport
  MTPA : Subsystem
  Sqrt : Sqrt
  Square : Math  Operator=square
  Square1 : Math  Operator=square
  Sum : Sum  Inputs=|++
  To Workspace1 : ToWorkspace  VariableName=id_pu_sim  SampleTime=ts_inv
      settings: MaxDataPoints=Ns_inv
  To Workspace2 : ToWorkspace  VariableName=iq_pu_sim  SampleTime=ts_inv
      settings: MaxDataPoints=Ns_inv
  To Workspace3 : ToWorkspace  VariableName=id_ref_pu_sim  SampleTime=ts_inv
      settings: MaxDataPoints=Ns_inv
  To Workspace4 : ToWorkspace  VariableName=iq_ref_pu_sim  SampleTime=ts_inv
      settings: MaxDataPoints=Ns_inv
  To Workspace5 : ToWorkspace  VariableName=ud_pu_sim  SampleTime=ts_inv
      settings: MaxDataPoints=Ns_inv
  To Workspace6 : ToWorkspace  VariableName=uq_pu_sim  SampleTime=ts_inv
      settings: MaxDataPoints=Ns_inv
  To Workspace7 : ToWorkspace  VariableName=u_mot_pu_sim  SampleTime=ts_inv
      settings: MaxDataPoints=Ns_inv
  dq_pi_with_vector_antiwindup : Subsystem
  id_ref : Subsystem
      settings: PortSchema="{\"entries\":[{\"content\":{\"sides\":[{\"content\":{},\"type\":\"ConnectorPlacement.EquallySpacedRectSide\",\"uuid\":\"42af5d69-f0eb-42c6-9e03-28c1d0757323\"},{\"content\":{\"connectorIds\":[\"Out1\"],\"side\":\"RIGHT\"},\"type\":\"ConnectorPlacement.EquallySpacedRectSide\",\"uuid\":\"dd68a9f9-d15f-4e57-9d9e-130889a7b90c\"},{\"content\":{\"connectorIds\":[\"In1\"],\"side\":\"TOP\"},\"type\":\"ConnectorPlacement.EquallySpacedRectSide\",\"uuid\":\"68c797a2-8439-4b8d-8368-b7485adf0676\"}]},\"type\":\"ConnectorPlacement.EquallySpacedConnector\",\"uuid\":\"693c5f1c-0580-4626-8f13-b27865dfb3ac\"}],\"packageUris\":[\"http://schema.mathworks.com/mf0/Connector/R2020b\"],\"version\":\"1.0\"}"
  idref/id : Scope  NumInputPorts=2
      settings: SampleTime=tc  ActiveDisplayYMinimum=-0.5383825399353187  ActiveDisplayYMaximum=0.059820282309629005
  iqref/iq : Scope  NumInputPorts=2
      settings: SampleTime=tc  ActiveDisplayYMinimum=-1.1641617765003931  ActiveDisplayYMaximum=0.12935130850004364  DataLoggingVariableName=ScopeData2
  ud : Outport
  uq : Outport  Port=2
  tag scope: id_pu_ref=global, iq_pu_ref=global, u_mot_pu_sim=global, ud_pu_sim=global, uq_pu_sim=global
  wires:
  [iq_pu] -> To Workspace2/1, iqref/iq/2, dq_pi_with_vector_antiwindup/4(iq)  "iq"
  [id_pu] -> To Workspace1/1, idref/id/2, dq_pi_with_vector_antiwindup/2(id)  "id"
  MTPA/1(Id_ref_mtpa) -> id_ref/1(id_mtpa), [id_pu_ref]  "id_ref"
  iq_ref/1 -> MTPA/1(iq_ref), To Workspace4/1, iqref/iq/1, dq_pi_with_vector_antiwindup/3(iq_ref), [iq_pu_ref]  "iq_ref"
  dq_pi_with_vector_antiwindup/1(ctrl_d_u) -> To Workspace5/1, [ud_pu_sim], Square1/1, ud/1
  dq_pi_with_vector_antiwindup/2(ctrl_q_u) -> [uq_pu_sim], To Workspace6/1, Square/1, uq/1
  Square/1 -> Sum/1
  Sum/1 -> Sqrt/1
  Square1/1 -> Sum/2
  Sqrt/1 -> [u_mot_pu_sim], To Workspace7/1
  id_ref/1(id_ref) -> To Workspace3/1, dq_pi_with_vector_antiwindup/1(id_ref), idref/id/1

== system afe_abc_inv_psm/afe_abc_inv_psm_mod1/inverter_control/current_ctrl/current_transformation ==
  u : Inport
  v : Inport  Port=2
  w : Inport  Port=3
  To Workspace2 : ToWorkspace  VariableName=ialpha_pu_sim  SampleTime=ts_inv
      settings: MaxDataPoints=Ns_inv
  To Workspace3 : ToWorkspace  VariableName=ibeta_pu_sim  SampleTime=ts_inv
      settings: MaxDataPoints=Ns_inv
  alphabeta2dq : MATLAB Function  TreatAsAtomicUnit=on  SystemSampleTime=ts_inv
  uvw2alphabeta : MATLAB Function  TreatAsAtomicUnit=on  SystemSampleTime=ts_inv
  tag scope: ialpha_pu=global, ibeta_pu=global, id_pu=global, iq_pu=global
  wires:
  w/1 -> uvw2alphabeta/3(w)
  alphabeta2dq/2(q) -> [iq_pu]  "iq_pu"
  alphabeta2dq/1(d) -> [id_pu]  "id_pu"
  v/1 -> uvw2alphabeta/2(v)
  uvw2alphabeta/2(beta) -> To Workspace3/1, [ibeta_pu], alphabeta2dq/2(beta)  "ibeta_pu"
  uvw2alphabeta/1(alpha) -> To Workspace2/1, [ialpha_pu], alphabeta2dq/1(alpha)  "ialpha_pu"
  [theta_hat] -> alphabeta2dq/3(gamma)
  u/1 -> uvw2alphabeta/1(u)

== system afe_abc_inv_psm/afe_abc_inv_psm_mod1/inverter_control/current_ctrl/sample_hold_normalization ==
  iu : Inport
  iv : Inport  Port=2
  iw : Inport  Port=3
  Gain : Gain  Gain=1/ibez
  Gain1 : Gain  Gain=1/ibez
  Gain2 : Gain  Gain=1/ibez
  Quantizer : Quantizer  QuantizationInterval=adc_quantization
  Quantizer1 : Quantizer  QuantizationInterval=adc_quantization
  Quantizer2 : Quantizer  QuantizationInterval=adc_quantization
  Unit Delay : UnitDelay  SampleTime=ts_inv  HasFrameUpgradeWarning=on
  Unit Delay1 : UnitDelay  SampleTime=ts_inv  HasFrameUpgradeWarning=on
  Unit Delay4 : UnitDelay  SampleTime=ts_inv  HasFrameUpgradeWarning=on
  Zero-Order Hold : ZeroOrderHold  SampleTime=ts_inv
  Zero-Order Hold1 : ZeroOrderHold  SampleTime=ts_inv
  Zero-Order Hold2 : ZeroOrderHold  SampleTime=ts_inv
  iu_pu : Outport
  iv_pu : Outport  Port=2
  iw_pu : Outport  Port=3
  wires:
  iu/1 -> Gain/1
  Zero-Order Hold1/1 -> Unit Delay1/1
  Zero-Order Hold2/1 -> Unit Delay4/1
  Zero-Order Hold/1 -> Unit Delay/1
  Unit Delay4/1 -> iw_pu/1
  Unit Delay1/1 -> iv_pu/1
  Unit Delay/1 -> iu_pu/1
  iw/1 -> Gain2/1
  iv/1 -> Gain1/1
  Gain2/1 -> Quantizer2/1
  Gain1/1 -> Quantizer1/1
  Gain/1 -> Quantizer/1
  Quantizer/1 -> Zero-Order Hold/1
  Quantizer1/1 -> Zero-Order Hold1/1
  Quantizer2/1 -> Zero-Order Hold2/1

== system afe_abc_inv_psm/grid/grid_emulator/breaker/switch_1 ==
  Switch : fl_lib/Electrical/Electrical Elements/Switch  R_closed=Ron Ohm  G_open=1e-8 1/Ohm  Threshold=7.5  i_specify=off  i_priority=None  i=0 A  i_nominal_specify=off  i_nominal_value=1  i_nominal_unit=A  v_specify=off  v_priority=None  v=0 V  v_nominal_specify=off  v_nominal_value=1  v_nominal_unit=V
  snubber : fl_lib/Electrical/Electrical Elements/Capacitor  c=Csnubber F  r=Rsnubber Ohm  g=0 1/Ohm  i_specify=off  i_priority=None  i=0 A  i_nominal_specify=off  i_nominal_value=1  i_nominal_unit=A  v_specify=off  v_priority=None  v=0 V  v_nominal_specify=off  v_nominal_value=1  v_nominal_unit=V  vc_specify=off  vc_priority=High  vc=0 V  vc_nominal_specify=off  vc_nominal_value=1  vc_nominal_unit=V
  G : PMIOPort  Side=Left
  C : PMIOPort  Port=2  Side=Left
  E : PMIOPort  Port=3  Side=Right
  connections:
  Switch/RConn2 -- snubber/LConn1 -- C/RConn1
  Switch/RConn1 -- G/RConn1
  Switch/LConn1 -- snubber/RConn1 -- E/RConn1
